simulink model "target_cam_robot_demo"  (Simulink 7.3)
settings: Solver=FixedStepDiscrete  SolverMode=SingleTasking  StartTime=0.0  StopTime=inf  RelTol=1e-3
PreLoadFcn:
  | waijung.modelPreload; % Required for working with Waijung Blockset. Do not remove.
undefined symbols (not defined in the file): A1, A2, A7, B10, B11, B12, C1, C2, C3, C4, C5, G14, H2, H3, H6, H7, HSEOSC, Link, LQFP176, ST, STM32F417IG
libraries: simulink x12, stm32f4_i2c_lib x8, stm32f4_tim_lib x2, stm32f4_io_lib x2, waijung_webserver x2, waijung_socket_lib x2, stm32f4_rcc_lib x1, stm32f4_device_config_lib x1, waijung_addon_module x1
(part 2 of 2)

== system target_cam_robot_demo/Camera OV7670/Init_/While Iterator_/Picture Size_/Subsystem/Subsystem ==
  Index : Inport
  Constant : Constant  Value=imgsize  OutDataType=fixdt(1, 16)  OutScaling=2^0
  Img120x160 : Subsystem  TreatAsAtomicUnit=on
  Img240x320 : Subsystem  TreatAsAtomicUnit=on
  Img480x640 : Subsystem  TreatAsAtomicUnit=on
  Merge_Count : Merge  Inputs=3
  Merge_Reg : Merge  Inputs=3
  Merge_Value : Merge  Inputs=3
  Switch Case : SwitchCase  CaseConditions={1,2}
  Count : Outport
  Reg : Outport  Port=2
  Value : Outport  Port=3
  wires:
  Switch Case/3 -> Img480x640/Action
  Constant/1 -> Switch Case/1
  Merge_Value/1 -> Value/1
  Merge_Reg/1 -> Reg/1
  Merge_Count/1 -> Count/1
  Index/1 -> Img480x640/1(Index), Img240x320/1(Index), Img120x160/1(Index)
  Img480x640/3(Value) -> Merge_Value/3
  Img240x320/3(Value) -> Merge_Value/2
  Img120x160/3(Value) -> Merge_Value/1
  Img480x640/2(Reg) -> Merge_Reg/3
  Img240x320/2(Reg) -> Merge_Reg/2
  Img120x160/2(Reg) -> Merge_Reg/1
  Img240x320/1(Count) -> Merge_Count/2
  Img480x640/1(Count) -> Merge_Count/3
  Img120x160/1(Count) -> Merge_Count/1
  Switch Case/2 -> Img240x320/Action
  Switch Case/1 -> Img120x160/Action

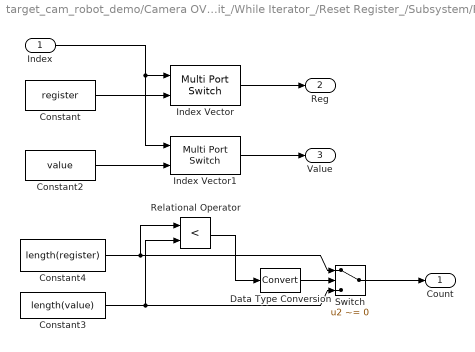
== system target_cam_robot_demo/Camera OV7670/Init_/While Iterator_/Reset Register_/Subsystem/Register List ==
  Index : Inport  OutDataType=fixdt(1, 16)  OutScaling=2^0
  Constant : Constant  Value=register  OutDataType=fixdt(1, 16)  OutScaling=2^0
  Constant2 : Constant  Value=value  OutDataType=fixdt(1, 16)  OutScaling=2^0
  Constant3 : Constant  Value=length(value)  OutDataType=fixdt(1, 16)  OutScaling=2^0
  Constant4 : Constant  Value=length(register)  OutDataType=fixdt(1, 16)  OutScaling=2^0
  Data Type Conversion : DataTypeConversion  OutDataType=fixdt(1, 16)  OutScaling=2^0
  Index Vector : MultiPortSwitch  Inputs=1  zeroidx=on  OutDataType=fixdt(1, 16)  OutScaling=2^0
  Index Vector1 : MultiPortSwitch  Inputs=1  zeroidx=on  OutDataType=fixdt(1, 16)  OutScaling=2^0
  Relational Operator : RelationalOperator  Operator=<  LogicOutDataTypeMode=boolean  LogicDataType=fixdt(0, 8)  OutDataTypeStr=boolean
  Switch : Switch  Criteria=u2 ~= 0  OutDataType=fixdt(1, 16)  OutScaling=2^0
  Count : Outport  OutDataType=fixdt(1, 16)  OutScaling=2^0
  Reg : Outport  Port=2  OutDataType=fixdt(1, 16)  OutScaling=2^0
  Value : Outport  Port=3  OutDataType=fixdt(1, 16)  OutScaling=2^0
  wires:
  Data Type Conversion/1 -> Switch/2
  Switch/1 -> Count/1
  Relational Operator/1 -> Data Type Conversion/1
  Constant3/1 -> Switch/3, Relational Operator/2
  Constant4/1 -> Switch/1, Relational Operator/1
  Index Vector1/1 -> Value/1
  Constant2/1 -> Index Vector1/2
  Index/1 -> Index Vector1/1, Index Vector/1
  Constant/1 -> Index Vector/2
  Index Vector/1 -> Reg/1

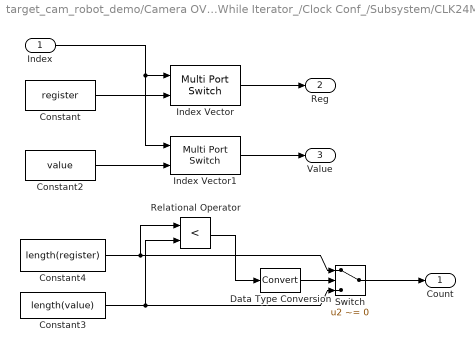
== system target_cam_robot_demo/Camera OV7670/Init_/While Iterator_/Clock Conf_/Subsystem/CLK24MHz_/Reg List_ ==
  Index : Inport  OutDataType=fixdt(1, 16)  OutScaling=2^0
  Constant : Constant  Value=register  OutDataType=fixdt(1, 16)  OutScaling=2^0
  Constant2 : Constant  Value=value  OutDataType=fixdt(1, 16)  OutScaling=2^0
  Constant3 : Constant  Value=length(value)  OutDataType=fixdt(1, 16)  OutScaling=2^0
  Constant4 : Constant  Value=length(register)  OutDataType=fixdt(1, 16)  OutScaling=2^0
  Data Type Conversion : DataTypeConversion  OutDataType=fixdt(1, 16)  OutScaling=2^0
  Index Vector : MultiPortSwitch  Inputs=1  zeroidx=on  OutDataType=fixdt(1, 16)  OutScaling=2^0
  Index Vector1 : MultiPortSwitch  Inputs=1  zeroidx=on  OutDataType=fixdt(1, 16)  OutScaling=2^0
  Relational Operator : RelationalOperator  Operator=<  LogicOutDataTypeMode=boolean  LogicDataType=fixdt(0, 8)  OutDataTypeStr=boolean
  Switch : Switch  Criteria=u2 ~= 0  OutDataType=fixdt(1, 16)  OutScaling=2^0
  Count : Outport  OutDataType=fixdt(1, 16)  OutScaling=2^0
  Reg : Outport  Port=2  OutDataType=fixdt(1, 16)  OutScaling=2^0
  Value : Outport  Port=3  OutDataType=fixdt(1, 16)  OutScaling=2^0
  wires:
  Data Type Conversion/1 -> Switch/2
  Switch/1 -> Count/1
  Relational Operator/1 -> Data Type Conversion/1
  Constant3/1 -> Switch/3, Relational Operator/2
  Constant4/1 -> Switch/1, Relational Operator/1
  Index Vector1/1 -> Value/1
  Constant2/1 -> Index Vector1/2
  Index/1 -> Index Vector1/1, Index Vector/1
  Constant/1 -> Index Vector/2
  Index Vector/1 -> Reg/1

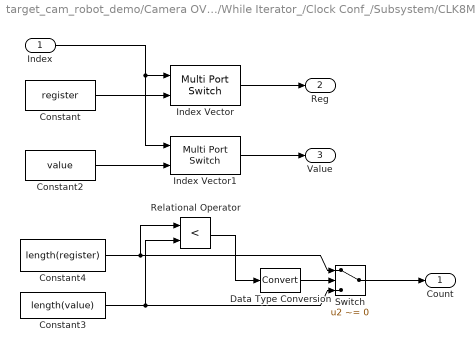
== system target_cam_robot_demo/Camera OV7670/Init_/While Iterator_/Clock Conf_/Subsystem/CLK8MHz_/Reg List_ ==
  Index : Inport  OutDataType=fixdt(1, 16)  OutScaling=2^0
  Constant : Constant  Value=register  OutDataType=fixdt(1, 16)  OutScaling=2^0
  Constant2 : Constant  Value=value  OutDataType=fixdt(1, 16)  OutScaling=2^0
  Constant3 : Constant  Value=length(value)  OutDataType=fixdt(1, 16)  OutScaling=2^0
  Constant4 : Constant  Value=length(register)  OutDataType=fixdt(1, 16)  OutScaling=2^0
  Data Type Conversion : DataTypeConversion  OutDataType=fixdt(1, 16)  OutScaling=2^0
  Index Vector : MultiPortSwitch  Inputs=1  zeroidx=on  OutDataType=fixdt(1, 16)  OutScaling=2^0
  Index Vector1 : MultiPortSwitch  Inputs=1  zeroidx=on  OutDataType=fixdt(1, 16)  OutScaling=2^0
  Relational Operator : RelationalOperator  Operator=<  LogicOutDataTypeMode=boolean  LogicDataType=fixdt(0, 8)  OutDataTypeStr=boolean
  Switch : Switch  Criteria=u2 ~= 0  OutDataType=fixdt(1, 16)  OutScaling=2^0
  Count : Outport  OutDataType=fixdt(1, 16)  OutScaling=2^0
  Reg : Outport  Port=2  OutDataType=fixdt(1, 16)  OutScaling=2^0
  Value : Outport  Port=3  OutDataType=fixdt(1, 16)  OutScaling=2^0
  wires:
  Index Vector/1 -> Reg/1
  Constant/1 -> Index Vector/2
  Index/1 -> Index Vector/1, Index Vector1/1
  Constant2/1 -> Index Vector1/2
  Index Vector1/1 -> Value/1
  Constant4/1 -> Relational Operator/1, Switch/1
  Constant3/1 -> Relational Operator/2, Switch/3
  Relational Operator/1 -> Data Type Conversion/1
  Switch/1 -> Count/1
  Data Type Conversion/1 -> Switch/2

== system target_cam_robot_demo/Camera OV7670/Init_/While Iterator_/Picture Size_/Subsystem/Subsystem/Img120x160 ==
  Index : Inport  OutDataType=fixdt(1, 16)  OutScaling=2^0
  Action Port : ActionPort  ActionType=case
  Register List : Subsystem  mask{register=uint8([58,61,140,64,18,50,23,24,25,26,3,12,62,112,113,114,115,162]), value=uint8([8,192,0,208,20,128,22,4,3,123,10,4,26,58,53,238,242,2])}
      mask prompts: register "Register Index"; value "Register Value"
      mask help:
      | Count:
      |  - Number of Register-Value pair.
      |  - Determine from lowest size, between Register and Value.
      | Reg:
      |  - Register index.
      | Value:
      |  - Data corresponding to specified register index.
  Count : Outport  OutDataType=fixdt(1, 16)  OutScaling=2^0
  Reg : Outport  Port=2  OutDataType=fixdt(1, 16)  OutScaling=2^0
  Value : Outport  Port=3  OutDataType=fixdt(1, 16)  OutScaling=2^0
  wires:
  Register List/3(Value) -> Value/1
  Register List/2(Reg) -> Reg/1
  Register List/1(Count) -> Count/1
  Index/1 -> Register List/1(Index)

== system target_cam_robot_demo/Camera OV7670/Init_/While Iterator_/Picture Size_/Subsystem/Subsystem/Img240x320 ==
  Index : Inport  OutDataType=fixdt(1, 16)  OutScaling=2^0
  Action Port : ActionPort  ActionType=case
  Register List : Subsystem  mask{register=uint8([58,61,140,64,18,50,23,24,25,26,3,12,62,112,113,114,115,162]), value=uint8([8,130,0,208,20,128,22,4,3,123,10,4,0,58,53,17,240,2])}
      mask prompts: register "Register Index"; value "Register Value"
      mask help:
      | Count:
      |  - Number of Register-Value pair.
      |  - Determine from lowest size, between Register and Value.
      | Reg:
      |  - Register index.
      | Value:
      |  - Data corresponding to specified register index.
  Count : Outport  OutDataType=fixdt(1, 16)  OutScaling=2^0
  Reg : Outport  Port=2  OutDataType=fixdt(1, 16)  OutScaling=2^0
  Value : Outport  Port=3  OutDataType=fixdt(1, 16)  OutScaling=2^0
  wires:
  Index/1 -> Register List/1(Index)
  Register List/1(Count) -> Count/1
  Register List/2(Reg) -> Reg/1
  Register List/3(Value) -> Value/1

== system target_cam_robot_demo/Camera OV7670/Init_/While Iterator_/Picture Size_/Subsystem/Subsystem/Img480x640 ==
  Index : Inport  OutDataType=fixdt(1, 16)  OutScaling=2^0
  Action Port : ActionPort  ActionType=default
  Register List : Subsystem  mask{register=uint8([58,61,140,64,18,50,23,24,25,26,3,12,62,112,113,114,115,162]), value=uint8([8,130,0,208,4,128,22,4,3,123,10,0,0,58,53,17,240,2])}
      mask prompts: register "Register Index"; value "Register Value"
      mask help:
      | Count:
      |  - Number of Register-Value pair.
      |  - Determine from lowest size, between Register and Value.
      | Reg:
      |  - Register index.
      | Value:
      |  - Data corresponding to specified register index.
  Count : Outport  OutDataType=fixdt(1, 16)  OutScaling=2^0
  Reg : Outport  Port=2  OutDataType=fixdt(1, 16)  OutScaling=2^0
  Value : Outport  Port=3  OutDataType=fixdt(1, 16)  OutScaling=2^0
  wires:
  Register List/3(Value) -> Value/1
  Register List/2(Reg) -> Reg/1
  Register List/1(Count) -> Count/1
  Index/1 -> Register List/1(Index)

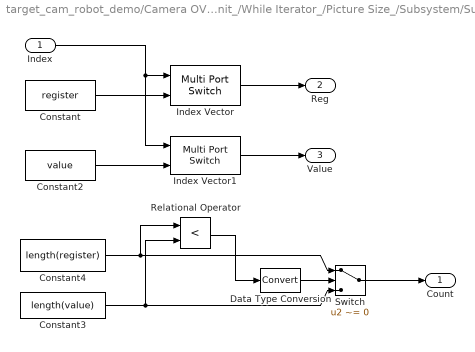
== system target_cam_robot_demo/Camera OV7670/Init_/While Iterator_/Picture Size_/Subsystem/Subsystem/Img120x160/Register List ==
  Index : Inport  OutDataType=fixdt(1, 16)  OutScaling=2^0
  Constant : Constant  Value=register  OutDataType=fixdt(1, 16)  OutScaling=2^0
  Constant2 : Constant  Value=value  OutDataType=fixdt(1, 16)  OutScaling=2^0
  Constant3 : Constant  Value=length(value)  OutDataType=fixdt(1, 16)  OutScaling=2^0
  Constant4 : Constant  Value=length(register)  OutDataType=fixdt(1, 16)  OutScaling=2^0
  Data Type Conversion : DataTypeConversion  OutDataType=fixdt(1, 16)  OutScaling=2^0
  Index Vector : MultiPortSwitch  Inputs=1  zeroidx=on  OutDataType=fixdt(1, 16)  OutScaling=2^0
  Index Vector1 : MultiPortSwitch  Inputs=1  zeroidx=on  OutDataType=fixdt(1, 16)  OutScaling=2^0
  Relational Operator : RelationalOperator  Operator=<  LogicOutDataTypeMode=boolean  LogicDataType=fixdt(0, 8)  OutDataTypeStr=boolean
  Switch : Switch  Criteria=u2 ~= 0  OutDataType=fixdt(1, 16)  OutScaling=2^0
  Count : Outport  OutDataType=fixdt(1, 16)  OutScaling=2^0
  Reg : Outport  Port=2  OutDataType=fixdt(1, 16)  OutScaling=2^0
  Value : Outport  Port=3  OutDataType=fixdt(1, 16)  OutScaling=2^0
  wires:
  Index Vector/1 -> Reg/1
  Constant/1 -> Index Vector/2
  Index/1 -> Index Vector/1, Index Vector1/1
  Constant2/1 -> Index Vector1/2
  Index Vector1/1 -> Value/1
  Constant4/1 -> Relational Operator/1, Switch/1
  Constant3/1 -> Relational Operator/2, Switch/3
  Relational Operator/1 -> Data Type Conversion/1
  Switch/1 -> Count/1
  Data Type Conversion/1 -> Switch/2

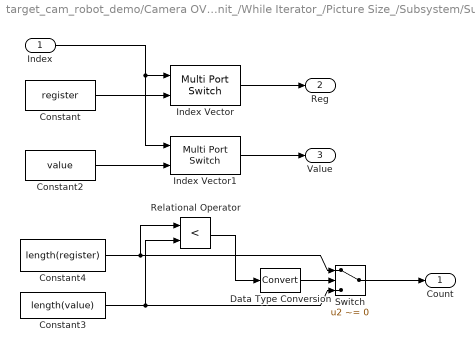
== system target_cam_robot_demo/Camera OV7670/Init_/While Iterator_/Picture Size_/Subsystem/Subsystem/Img240x320/Register List ==
  Index : Inport  OutDataType=fixdt(1, 16)  OutScaling=2^0
  Constant : Constant  Value=register  OutDataType=fixdt(1, 16)  OutScaling=2^0
  Constant2 : Constant  Value=value  OutDataType=fixdt(1, 16)  OutScaling=2^0
  Constant3 : Constant  Value=length(value)  OutDataType=fixdt(1, 16)  OutScaling=2^0
  Constant4 : Constant  Value=length(register)  OutDataType=fixdt(1, 16)  OutScaling=2^0
  Data Type Conversion : DataTypeConversion  OutDataType=fixdt(1, 16)  OutScaling=2^0
  Index Vector : MultiPortSwitch  Inputs=1  zeroidx=on  OutDataType=fixdt(1, 16)  OutScaling=2^0
  Index Vector1 : MultiPortSwitch  Inputs=1  zeroidx=on  OutDataType=fixdt(1, 16)  OutScaling=2^0
  Relational Operator : RelationalOperator  Operator=<  LogicOutDataTypeMode=boolean  LogicDataType=fixdt(0, 8)  OutDataTypeStr=boolean
  Switch : Switch  Criteria=u2 ~= 0  OutDataType=fixdt(1, 16)  OutScaling=2^0
  Count : Outport  OutDataType=fixdt(1, 16)  OutScaling=2^0
  Reg : Outport  Port=2  OutDataType=fixdt(1, 16)  OutScaling=2^0
  Value : Outport  Port=3  OutDataType=fixdt(1, 16)  OutScaling=2^0
  wires:
  Data Type Conversion/1 -> Switch/2
  Switch/1 -> Count/1
  Relational Operator/1 -> Data Type Conversion/1
  Constant3/1 -> Switch/3, Relational Operator/2
  Constant4/1 -> Switch/1, Relational Operator/1
  Index Vector1/1 -> Value/1
  Constant2/1 -> Index Vector1/2
  Index/1 -> Index Vector1/1, Index Vector/1
  Constant/1 -> Index Vector/2
  Index Vector/1 -> Reg/1

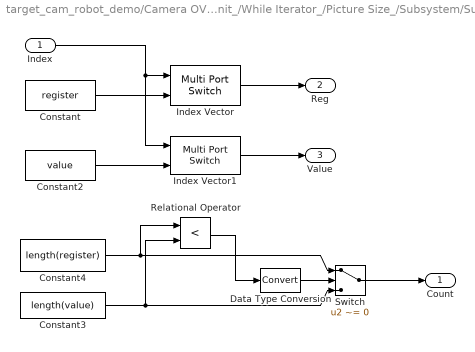
== system target_cam_robot_demo/Camera OV7670/Init_/While Iterator_/Picture Size_/Subsystem/Subsystem/Img480x640/Register List ==
  Index : Inport  OutDataType=fixdt(1, 16)  OutScaling=2^0
  Constant : Constant  Value=register  OutDataType=fixdt(1, 16)  OutScaling=2^0
  Constant2 : Constant  Value=value  OutDataType=fixdt(1, 16)  OutScaling=2^0
  Constant3 : Constant  Value=length(value)  OutDataType=fixdt(1, 16)  OutScaling=2^0
  Constant4 : Constant  Value=length(register)  OutDataType=fixdt(1, 16)  OutScaling=2^0
  Data Type Conversion : DataTypeConversion  OutDataType=fixdt(1, 16)  OutScaling=2^0
  Index Vector : MultiPortSwitch  Inputs=1  zeroidx=on  OutDataType=fixdt(1, 16)  OutScaling=2^0
  Index Vector1 : MultiPortSwitch  Inputs=1  zeroidx=on  OutDataType=fixdt(1, 16)  OutScaling=2^0
  Relational Operator : RelationalOperator  Operator=<  LogicOutDataTypeMode=boolean  LogicDataType=fixdt(0, 8)  OutDataTypeStr=boolean
  Switch : Switch  Criteria=u2 ~= 0  OutDataType=fixdt(1, 16)  OutScaling=2^0
  Count : Outport  OutDataType=fixdt(1, 16)  OutScaling=2^0
  Reg : Outport  Port=2  OutDataType=fixdt(1, 16)  OutScaling=2^0
  Value : Outport  Port=3  OutDataType=fixdt(1, 16)  OutScaling=2^0
  wires:
  Index Vector/1 -> Reg/1
  Constant/1 -> Index Vector/2
  Index/1 -> Index Vector/1, Index Vector1/1
  Constant2/1 -> Index Vector1/2
  Index Vector1/1 -> Value/1
  Constant4/1 -> Relational Operator/1, Switch/1
  Constant3/1 -> Relational Operator/2, Switch/3
  Relational Operator/1 -> Data Type Conversion/1
  Switch/1 -> Count/1
  Data Type Conversion/1 -> Switch/2
